simulink model "Quater_passive"  (Simulink 6.3)
settings: Solver=ode45  StartTime=0.0  StopTime=10.0  RelTol=1e-3
settings Model: LastModifiedBy=angel  StrictBusMsg=None
settings OptimizationCC: BooleanDataType=off
settings DebuggingCC: SolverPrmCheckMsg=none
settings HardwareCC: TargetUnknown=on

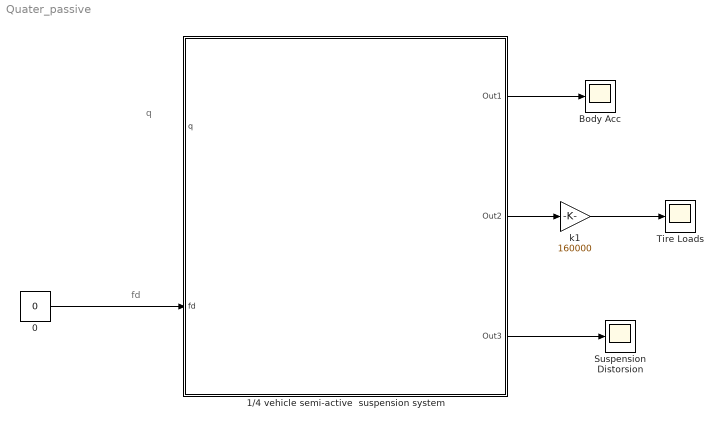
== system Quater_passive ==
  note: q
  note: fd
  0 : Constant  Value=0
  1/4 vehicle semi-active  suspension system : Subsystem
      mask Display: image(imread('Semi_acitve model2DOF.jpg'));
  Body Acc : Scope
      settings: YMin=-1.75  YMax=3.75
  Suspension Distorsion : Scope
      settings: SaveName=ScopeData2
  Tire Loads : Scope
  k1 : Gain  Gain=160000  SaturateOnIntegerOverflow=on
  wires:
  ? -> 1/4 vehicle semi-active  suspension system/1(q)
  1/4 vehicle semi-active  suspension system/1(Out1) -> Body Acc/1
  1/4 vehicle semi-active  suspension system/3(Out3) -> Suspension Distorsion/1
  1/4 vehicle semi-active  suspension system/2(Out2) -> k1/1
  k1/1 -> Tire Loads/1
  0/1 -> 1/4 vehicle semi-active  suspension system/2(fd)

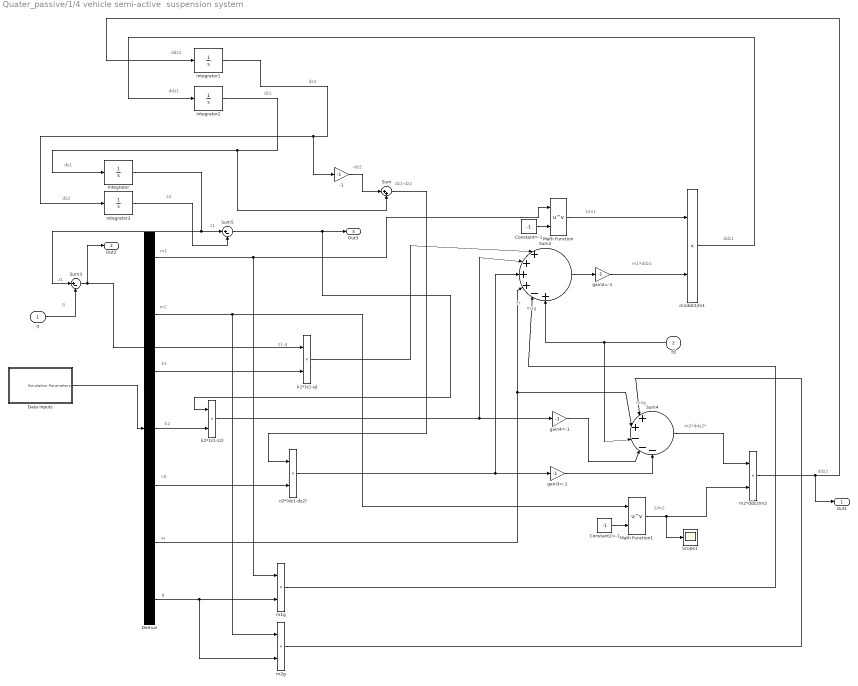
== system Quater_passive/1/4 vehicle semi-active  suspension system ==
  note: m1
  note: k1
  note: m2
  note: k2
  note: c0
  note: z1
  note: dz1
  note: Fr
  note: g
  note: dz2
  note: -dz2
  note: dz1-dz2
  note: dz1
  note: dz2
  note: ddz2
  note: q
  note: z1
  note: z1-q
  note: Fr
  note: m1g
  note: m1*ddz1
  note: 1/m1
  note: ddz1
  note: m2g
  note: m2*ddz2*
  note: 1/m2
  note: ddz2
  note: z2
  note: ddz1
  q : Inport
  fd : Inport  Orientation=left  Port=2
  -1 : Gain  Gain=-1  SaturateOnIntegerOverflow=on
  Constant2=-1 : Constant  Value=-1
  Constant=-1 : Constant  Value=-1
  Data Inputs : Subsystem
  Demux : Demux  Outputs=7  BusSelectionMode=on
  Integrator{,1..3} (4 alike) : Integrator
  Math Function : Math  Operator=pow  SaturateOnIntegerOverflow=on
  Math Function1 : Math  Operator=pow  SaturateOnIntegerOverflow=on
  Scope1 : Scope
      settings: SaveName=ScopeData5
  Sum : Sum  Inputs=|++  SaturateOnIntegerOverflow=on  InputSameDT=on
  Sum2 : Sum  Inputs=|++++-+  SaturateOnIntegerOverflow=on  InputSameDT=on
  Sum3 : Sum  Inputs=|+-  SaturateOnIntegerOverflow=on  InputSameDT=on
  Sum4 : Sum  Inputs=|++---  SaturateOnIntegerOverflow=on  InputSameDT=on
  Sum5 : Sum  Inputs=|+-  SaturateOnIntegerOverflow=on  InputSameDT=on
  c0*(dz1-dz2) : Product  SaturateOnIntegerOverflow=on  RndMeth=Zero  InputSameDT=on
  gain2=-1 : Gain  Gain=-1  SaturateOnIntegerOverflow=on
  gain3=-1 : Gain  Gain=-1  SaturateOnIntegerOverflow=on
  gain4=-1 : Gain  Gain=-1  SaturateOnIntegerOverflow=on
  k1*(z1-q) : Product  SaturateOnIntegerOverflow=on  RndMeth=Zero  InputSameDT=on
  k2*(z1-z2) : Product  SaturateOnIntegerOverflow=on  RndMeth=Zero  InputSameDT=on
  m1ddz1/m1 : Product  SaturateOnIntegerOverflow=on  RndMeth=Zero  InputSameDT=on
  m1g : Product  SaturateOnIntegerOverflow=on  RndMeth=Zero  InputSameDT=on
  m2*ddz2/m2 : Product  SaturateOnIntegerOverflow=on  RndMeth=Zero  InputSameDT=on
  m2g : Product  SaturateOnIntegerOverflow=on  RndMeth=Zero  InputSameDT=on
  Out1 : Outport
  Out2 : Outport  Port=2
  Out3 : Outport  Port=3
  wires:
  Data Inputs/1("Simulaiton Parameters ") -> Demux/1
  Demux/1 -> m1g/1, Math Function/1
  Integrator2/1 -> Sum/2, Integrator/1
  Integrator/1 -> Sum5/1, Sum3/1
  Demux/5 -> c0*(dz1-dz2)/2
  -1/1 -> Sum/1
  Sum/1 -> c0*(dz1-dz2)/1
  Integrator1/1 -> -1/1, Integrator3/1
  Demux/4 -> k2*(z1-z2)/2
  Demux/3 -> k1*(z1-q)/2
  Sum3/1 -> k1*(z1-q)/1, Out2/1
  Sum2/1 -> gain2=-1/1
  gain2=-1/1 -> m1ddz1/m1/2
  k1*(z1-q)/1 -> Sum2/1
  k2*(z1-z2)/1 -> Sum2/2, gain4=-1/1
  c0*(dz1-dz2)/1 -> Sum2/3, gain3=-1/1
  fd/1 -> Sum2/6, Sum4/3
  Constant=-1/1 -> Math Function/2
  Math Function/1 -> m1ddz1/m1/1
  m1ddz1/m1/1 -> Integrator2/1
  Demux/6 -> Sum2/4, Sum4/2
  gain3=-1/1 -> Sum4/5
  gain4=-1/1 -> Sum4/4
  Sum4/1 -> m2*ddz2/m2/1
  Demux/7 -> m1g/2, m2g/2
  Demux/2 -> m2g/1, Math Function1/1
  m1g/1 -> Sum2/5
  m2g/1 -> Sum4/1
  Constant2=-1/1 -> Math Function1/2
  Math Function1/1 -> m2*ddz2/m2/2, Scope1/1
  m2*ddz2/m2/1 -> Integrator1/1, Out1/1
  Integrator3/1 -> Sum5/2
  Sum5/1 -> k2*(z1-z2)/1, Out3/1
  q/1 -> Sum3/2

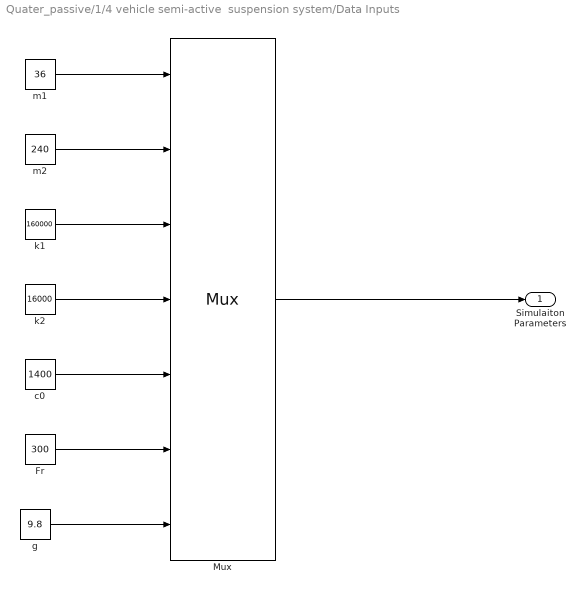
== system Quater_passive/1/4 vehicle semi-active  suspension system/Data Inputs ==
  Fr : Constant  Value=300
  Mux : Mux  Inputs=7
  c0 : Constant  Value=1400
  g : Constant  Value=9.8
  k1 : Constant  Value=160000
  k2 : Constant  Value=16000
  m1 : Constant  Value=36
  m2 : Constant  Value=240
  "Simulaiton Parameters " : Outport
  wires:
  m1/1 -> Mux/1
  m2/1 -> Mux/2
  k1/1 -> Mux/3
  k2/1 -> Mux/4
  c0/1 -> Mux/5
  Fr/1 -> Mux/6
  g/1 -> Mux/7
  Mux/1 -> "Simulaiton Parameters "/1
